simulink model "Adaptive_Control_Kd"  (R2021b)
settings: Solver=VariableStepAuto  StartTime=0.0  StopTime=50  RelTol=1e-3
undefined symbols (not defined in the file or in its folder): Kd, Kpi, Lambda, q_dq_init
(part 3 of 4)

== matlab function Adaptive_Control_Kd/Robot ==
  data: q_dq input; dq_ddq output; u input; q output; dq output
function [dq_ddq,q,dq] = fcn(q_dq,u)
    q = q_dq(1:length(q_dq)/2);
    dq = q_dq(length(q_dq)/2+1:length(q_dq));
    g_num = -9.81;

    in1 = q;
    in2 = [q;dq];
    in3 = [q;g_num];
%     in1 = mat2cell(in1,ones(numel(in1),1),1);
%     in2 = mat2cell(in2,ones(numel(in2),1),1);
%     in3 = mat2cell(in3,ones(numel(in3),1),1);


    M = M_fun(in1(1),in1(2),in1(3),in1(4),in1(5),in1(6));
    C = C_fun(in2(1),in2(2),in2(3),in2(4),in2(5),in2(6),in2(7),in2(8),in2(9),in2(10),in2(11),in2(12));
    G = G_fun(in3(1),in3(2),in3(3),in3(4),in3(5),in3(6),in3(7));

    ddq = M\(u - C - G);
    
    dq_ddq = [dq;ddq];

end
